simulink subsystem "F550_ControlAllocation_sub"  (R2024a)
settings: Solver=VariableStepAuto  StartTime=0.0  StopTime=10.0  RelTol=1e-3
settings Model: Creator=CNU_UASG  LastModifiedBy=CNU_UASG

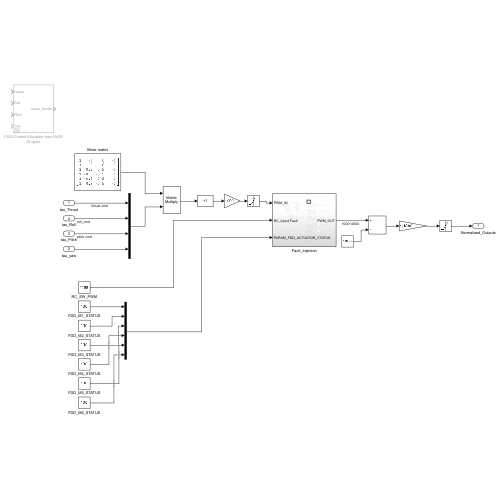
[thumbnail: Simulink's stored preview of the top-level diagram]
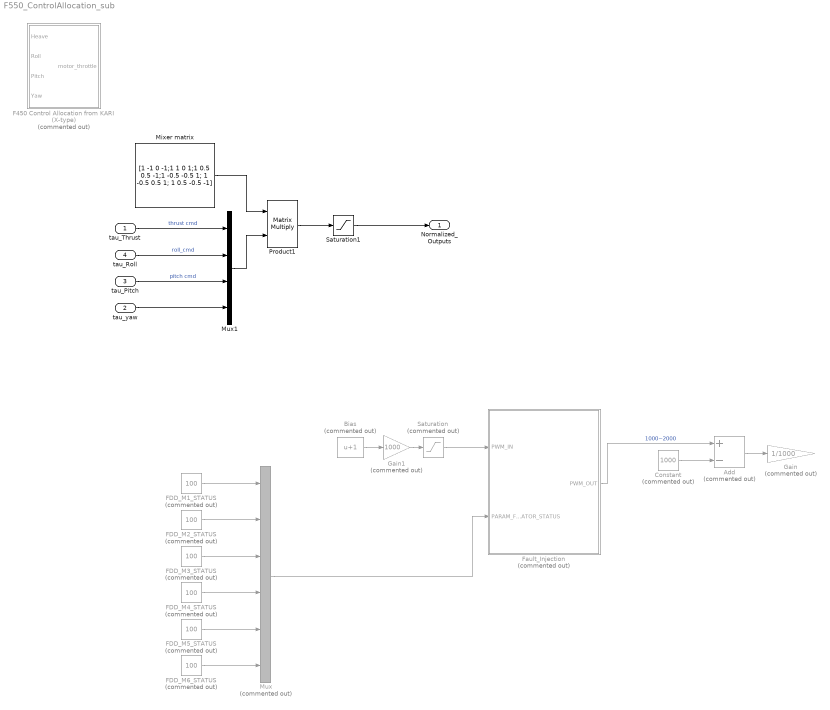
== system F550_ControlAllocation_sub ==
  tau_Thrust : Inport
  tau_yaw : Inport  Port=2
  tau_Pitch : Inport  Port=3
  tau_Roll : Inport  Port=4
  Add : Sum  Commented=on  Inputs=+-
  Bias : Bias  Commented=on  Bias=1  SaturateOnIntegerOverflow=off
  Constant : Constant  Commented=on  Value=1000
  F450 Control Allocation from KARI (X-type) : Subsystem  Commented=on
  FDD_M1_STATUS : Constant  Commented=on  Value=100
  FDD_M2_STATUS : Constant  Commented=on  Value=100
  FDD_M3_STATUS : Constant  Commented=on  Value=100
  FDD_M4_STATUS : Constant  Commented=on  Value=100
  FDD_M5_STATUS : Constant  Commented=on  Value=100
  FDD_M6_STATUS : Constant  Commented=on  Value=100
  Fault_Injection : Subsystem  Commented=on  VariantControl=(default)
  Gain : Gain  Commented=on  Gain=1/1000
  Gain1 : Gain  Commented=on  Gain=1000  OutDataTypeStr=uint16
  Mixer matrix : Constant  Value=[1 -1 0 -1;1 1 0 1;1 0.5 0.5 -1;1 -0.5 -0.5 1; 1 -0.5 0.5 1; 1 0.5 -0.5 -1]  OutDataTypeStr=Inherit: Inherit via back propagation  SampleTime=-1
  Mux : Mux  Commented=on  Inputs=6
  Mux1 : Mux
  Product1 : Product  Multiplication=Matrix(*)  RndMeth=Zero
  Saturation : Saturate  Commented=on  UpperLimit=2000  LowerLimit=1000  LinearizeAsGain=off
  Saturation1 : Saturate  UpperLimit=1  LowerLimit=0  LinearizeAsGain=off
  Normalized_Outputs : Outport
  wires:
  FDD_M1_STATUS/1 -> Mux/1
  FDD_M3_STATUS/1 -> Mux/3
  FDD_M2_STATUS/1 -> Mux/2
  Mux/1 -> Fault_Injection/2(PARAM_FDD_ACTUATOR_STATUS)
  FDD_M6_STATUS/1 -> Mux/6
  Bias/1 -> Gain1/1
  tau_Pitch/1 -> Mux1/3  "pitch cmd"
  Saturation/1 -> Fault_Injection/1(PWM_IN)
  Add/1 -> Gain/1
  Fault_Injection/1(PWM_OUT) -> Add/1  "1000~2000"
  FDD_M5_STATUS/1 -> Mux/5
  tau_Thrust/1 -> Mux1/1  "thrust cmd"
  Gain1/1 -> Saturation/1
  FDD_M4_STATUS/1 -> Mux/4
  Constant/1 -> Add/2
  tau_yaw/1 -> Mux1/4
  Mixer matrix/1 -> Product1/1
  tau_Roll/1 -> Mux1/2  "roll_cmd"
  Mux1/1 -> Product1/2
  Saturation1/1 -> Normalized_Outputs/1
  Product1/1 -> Saturation1/1

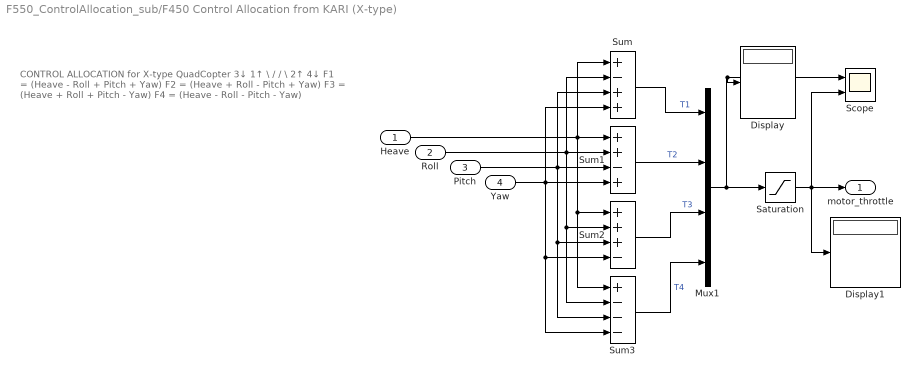
== system F550_ControlAllocation_sub/F450 Control Allocation from KARI (X-type) ==
  note: CONTROL ALLOCATION for X-type QuadCopter
      | 3↓ 1↑
      | \ /
      | / \
      | 2↑ 4↓
      | F1 = (Heave - Roll + Pitch + Yaw)
      | F2 = (Heave + Roll - Pitch + Yaw)
      | F3 = (Heave + Roll + Pitch - Yaw)
      | F4 = (Heave - Roll - Pitch - Yaw)
  Heave : Inport
  Roll : Inport  Port=2
  Pitch : Inport  Port=3
  Yaw : Inport  Port=4
  Display : Display
  Display1 : Display
  Mux1 : Mux
  Saturation : Saturate  UpperLimit=1  LowerLimit=0
      settings: AttributesFormatString=%<LowerLimit>~%<UpperLimit>
  Scope : Scope  NumInputPorts=2
  Sum : Sum  Inputs=+-++
  Sum1 : Sum  Inputs=++-+
  Sum2 : Sum  Inputs=+++-
  Sum3 : Sum  Inputs=+---
  motor_throttle : Outport
  wires:
  Sum2/1 -> Mux1/3  "T3"
  Sum/1 -> Mux1/1  "T1"
  Heave/1 -> Sum1/1, Sum/1, Sum2/1, Sum3/1
  Roll/1 -> Sum1/2, Sum/2, Sum2/2, Sum3/2
  Sum1/1 -> Mux1/2  "T2"
  Mux1/1 -> Display/1, Scope/1, Saturation/1
  Sum3/1 -> Mux1/4  "T4"
  Pitch/1 -> Sum1/3, Sum/3, Sum2/3, Sum3/3
  Yaw/1 -> Sum1/4, Sum/4, Sum2/4, Sum3/4
  Saturation/1 -> Display1/1, Scope/2, motor_throttle/1

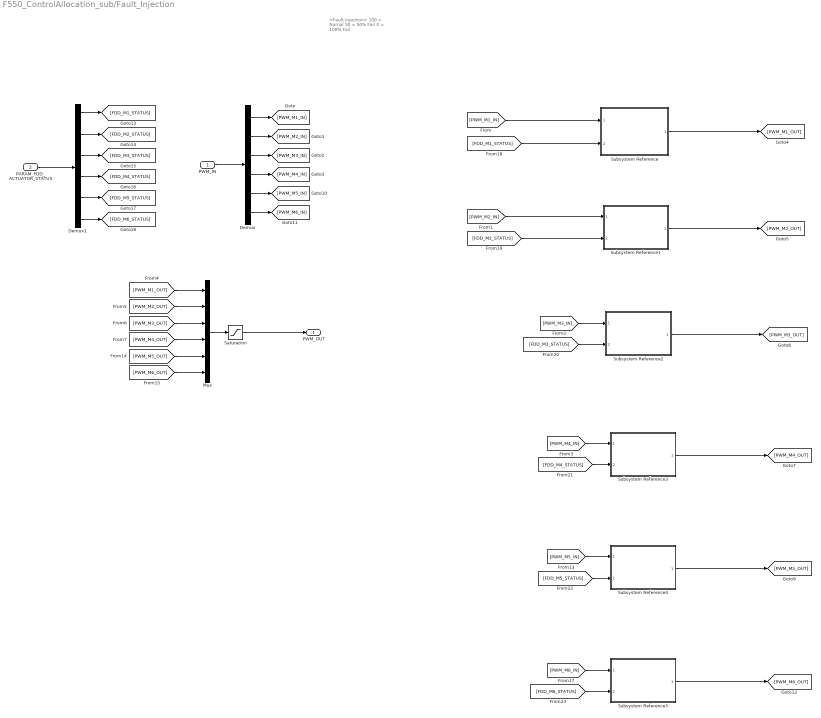
== system F550_ControlAllocation_sub/Fault_Injection ==
  note: <Fault Injection>
      | 100 = Nornal
      | 50 = 50% Fail
      | 0 = 100% Fail
  PWM_IN : Inport
  PARAM_FDD_ACTUATOR_STATUS : Inport  Port=2
  Demux : Demux  Outputs=6
  Demux1 : Demux  Outputs=6
  Mux : Mux  Inputs=6
  Saturation : Saturate  UpperLimit=2000  LowerLimit=1000
  Subsystem Reference{,1..5} (6 alike) : Subsystem  ReferencedSubsystem=F550_calcFaultInjectedPWM
  PWM_OUT : Outport
  wires:
  [FDD_M6_STATUS] -> Subsystem Reference5/2
  [FDD_M5_STATUS] -> Subsystem Reference4/2
  [FDD_M4_STATUS] -> Subsystem Reference3/2
  [FDD_M3_STATUS] -> Subsystem Reference2/2
  [FDD_M2_STATUS] -> Subsystem Reference1/2
  [FDD_M1_STATUS] -> Subsystem Reference/2
  Demux/1 -> [PWM_M1_IN]
  Demux/2 -> [PWM_M2_IN]
  Demux/3 -> [PWM_M3_IN]
  Demux/4 -> [PWM_M4_IN]
  [PWM_M1_IN] -> Subsystem Reference/1
  [PWM_M2_IN] -> Subsystem Reference1/1
  [PWM_M3_IN] -> Subsystem Reference2/1
  [PWM_M4_IN] -> Subsystem Reference3/1
  [PWM_M1_OUT] -> Mux/1
  [PWM_M2_OUT] -> Mux/2
  [PWM_M3_OUT] -> Mux/3
  [PWM_M4_OUT] -> Mux/4
  [PWM_M5_IN] -> Subsystem Reference4/1
  Demux/5 -> [PWM_M5_IN]
  Demux/6 -> [PWM_M6_IN]
  [PWM_M5_OUT] -> Mux/5
  [PWM_M6_OUT] -> Mux/6
  [PWM_M6_IN] -> Subsystem Reference5/1
  Subsystem Reference/1 -> [PWM_M1_OUT]
  Subsystem Reference1/1 -> [PWM_M2_OUT]
  Subsystem Reference2/1 -> [PWM_M3_OUT]
  Subsystem Reference3/1 -> [PWM_M4_OUT]
  Subsystem Reference4/1 -> [PWM_M5_OUT]
  Subsystem Reference5/1 -> [PWM_M6_OUT]
  PWM_IN/1 -> Demux/1
  Mux/1 -> Saturation/1
  PARAM_FDD_ACTUATOR_STATUS/1 -> Demux1/1
  Demux1/1 -> [FDD_M1_STATUS]
  Demux1/2 -> [FDD_M2_STATUS]
  Demux1/3 -> [FDD_M3_STATUS]
  Demux1/4 -> [FDD_M4_STATUS]
  Demux1/5 -> [FDD_M5_STATUS]
  Demux1/6 -> [FDD_M6_STATUS]
  Saturation/1 -> PWM_OUT/1
